simulink model "autoMBD_example_PI_MultirateTrigger"  (R2020b)
settings: Solver=FixedStepAuto  StartTime=0.0  StopTime=10.0  FixedStep=0.0001  RelTol=1e-3
undefined symbols (not defined in the file): DiscIntNeverNeededParam
settings Model: Creator=k  LastModifiedBy=k
settings OptimizationCC: DefaultParameterBehavior=Inlined  EnhancedBackFolding=on  PassReuseOutputArgsAs=Individual arguments  ZeroExternalMemoryAtStartup=off  ZeroInternalMemoryAtStartup=off  OptimizeBlockOrder=speed  DifferentSizesBufferReuse=on  OptimizationCustomize=off  EfficientTunableParamExpr=on
settings DebuggingCC: ParameterTunabilityLossMsg=error
settings SFSimCC: MATLABDynamicMemAlloc=off
settings RTWCC: Description=Embedded Coder  SystemTargetFile=ert.tlc  GenCodeOnly=on  TemplateMakefile=ert_default_tmf
settings CodeAppCC: ForceParamTrailComments=on  IgnoreCustomStorageClasses=off  OperatorAnnotations=on  SimulinkDataObjDesc=on  SFDataObjDesc=on  InsertBlockDesc=on
settings ERTTargetCC: TargetLangStandard=C99 (ISO)  GenerateSampleERTMain=on  InlinedParameterPlacement=NonHierarchical  ERTCustomFileTemplate=example_file_process.tlc

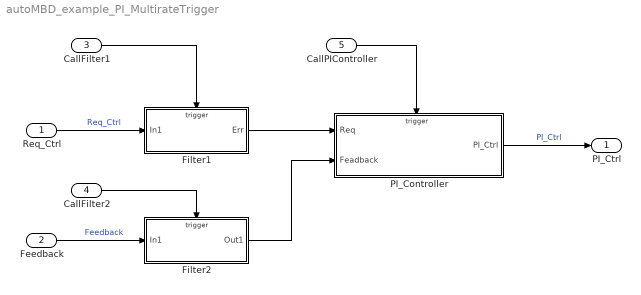
== system autoMBD_example_PI_MultirateTrigger ==
  Req_Ctrl : Inport
  Feedback : Inport  Port=2
  CallFilter1 : Inport  Port=3  OutputFunctionCall=on
  CallFilter2 : Inport  Port=4  OutputFunctionCall=on
  CallPIController : Inport  Port=5  SampleTime=0.001  OutputFunctionCall=on
  Filter1 : Subsystem  TreatAsAtomicUnit=on  RTWFcnName=Filter1
      settings: RTWFcnNameOpts=User specified
  Filter2 : Subsystem  TreatAsAtomicUnit=on  RTWFcnName=Filter2
      settings: RTWFcnNameOpts=User specified
  PI_Controller : Subsystem  TreatAsAtomicUnit=on  SystemSampleTime=0.001  RTWFcnName=PI_Controller
      settings: RTWFcnNameOpts=User specified
  PI_Ctrl : Outport
  wires:
  Req_Ctrl/1 -> Filter1/1(In1)  "Req_Ctrl"
  Feedback/1 -> Filter2/1(In1)  "Feedback"
  Filter1/1(Err) -> PI_Controller/1(Req)
  PI_Controller/1(PI_Ctrl) -> PI_Ctrl/1  "PI_Ctrl"
  Filter2/1(Out1) -> PI_Controller/2(Feadback)
  CallFilter1/1 -> Filter1/Trigger
  CallFilter2/1 -> Filter2/Trigger
  CallPIController/1 -> PI_Controller/Trigger

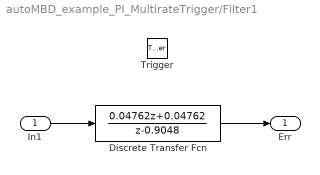
== system autoMBD_example_PI_MultirateTrigger/Filter1 ==
  In1 : Inport
  Trigger : TriggerPort  TriggerType=function-call  VariantControl=Variant  PortDimensions=1
  Discrete Transfer Fcn : DiscreteTransferFcn  Numerator=[0.04762 0.04762]  Denominator=[1 -0.9048]
  Err : Outport
  wires:
  In1/1 -> Discrete Transfer Fcn/1
  Discrete Transfer Fcn/1 -> Err/1

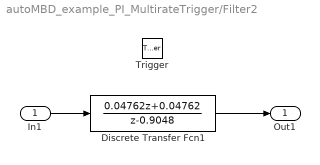
== system autoMBD_example_PI_MultirateTrigger/Filter2 ==
  In1 : Inport
  Trigger : TriggerPort  TriggerType=function-call  VariantControl=Variant  PortDimensions=1
  Discrete Transfer Fcn1 : DiscreteTransferFcn  Numerator=[0.04762 0.04762]  Denominator=[1 -0.9048]
  Out1 : Outport
  wires:
  In1/1 -> Discrete Transfer Fcn1/1
  Discrete Transfer Fcn1/1 -> Out1/1

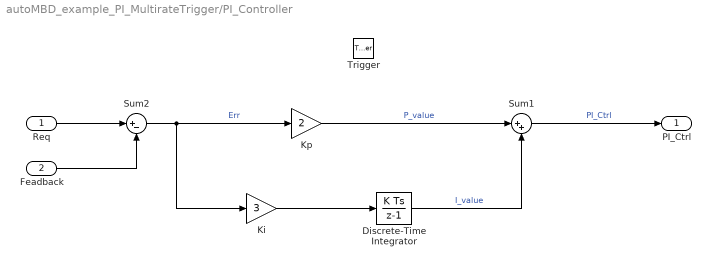
== system autoMBD_example_PI_MultirateTrigger/PI_Controller ==
  Req : Inport
  Feadback : Inport  Port=2
  Trigger : TriggerPort  TriggerType=function-call  VariantControl=Variant  SampleTimeType=periodic  SampleTime=-1  PortDimensions=1
  Discrete-Time Integrator : DiscreteIntegrator  SampleTime=-1  ICPrevOutput=DiscIntNeverNeededParam  ICPrevScaledInput=DiscIntNeverNeededParam
  Ki : Gain  Gain=3
  Kp : Gain  Gain=2
  Sum1 : Sum  Inputs=|++
  Sum2 : Sum  Inputs=|+-
  PI_Ctrl : Outport
  wires:
  Sum1/1 -> PI_Ctrl/1  "PI_Ctrl"
  Sum2/1 -> Ki/1, Kp/1  "Err"
  Discrete-Time Integrator/1 -> Sum1/2  "I_value"
  Ki/1 -> Discrete-Time Integrator/1
  Kp/1 -> Sum1/1  "P_value"
  Req/1 -> Sum2/1
  Feadback/1 -> Sum2/2
